simulink model "Environment"  (R2014b)
settings: Solver=ode45  StartTime=0.0  StopTime=10.0  RelTol=1e-3
model workspace (MATLAB code in the model file):
  | switch(Env)
  |    case 'Pikes Peak'
  |       load Evn_Pikes_Peak;
  |    case 'IOM'
  |       load Evn_IOM;
  |    otherwise
  |       load Environment
  | end
undefined symbols (not defined in the file): altx, alty, g, L, M, P0, R, Rcx, Rcy, T0
settings Model: Creator=Nathan  LastModifiedBy=Nathan
settings DebuggingCC: UnderspecifiedInitializationDetection=Classic  MergeDetectMultiDrivingBlocksExec=none  StateNameClashWarn=warning

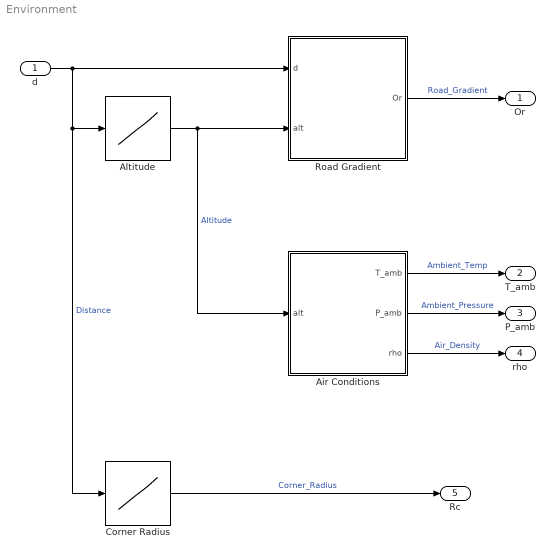
== system Environment ==
  d : Inport
  Air Conditions : Subsystem
  Altitude : Lookup_n-D  NumberOfTableDimensions=1  BreakpointsForDimension1=altx  Table=alty  ExtrapMethod=Clip  DiagnosticForOutOfRangeInput=Warning  UseLastTableValue=on  RndMeth=Simplest  InputSameDT=on
  Corner Radius : Lookup_n-D  NumberOfTableDimensions=1  BreakpointsForDimension1=Rcx  Table=Rcy  ExtrapMethod=Clip  DiagnosticForOutOfRangeInput=Warning  UseLastTableValue=on  RndMeth=Simplest  InputSameDT=on
  Road Gradient : Subsystem
  Or : Outport
  T_amb : Outport  Port=2
  P_amb : Outport  Port=3
  rho : Outport  Port=4
  Rc : Outport  Port=5
  wires:
  d/1 -> Road Gradient/1(d), Corner Radius/1, Altitude/1  "Distance"
  Road Gradient/1(Or) -> Or/1  "Road_Gradient"
  Altitude/1 -> Air Conditions/1(alt), Road Gradient/2(alt)  "Altitude"
  Air Conditions/1("T_amb ") -> T_amb/1  "Ambient_Temp"
  Air Conditions/2(P_amb) -> P_amb/1  "Ambient_Pressure"
  Air Conditions/3(rho) -> rho/1  "Air_Density"
  Corner Radius/1 -> Rc/1  "Corner_Radius"

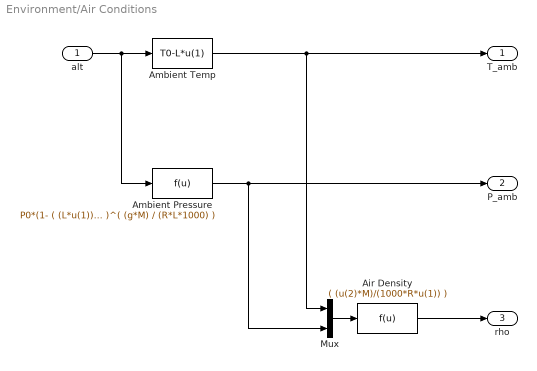
== system Environment/Air Conditions ==
  alt : Inport
  Air Density : Fcn  Expr=( (u(2)*M)/(1000*R*u(1)) )
  Ambient Pressure : Fcn  Expr=P0*(1- ( (L*u(1))/(T0) ) )^( (g*M) / (R*L*1000) )
  Ambient Temp : Fcn  Expr=T0-L*u(1)
  Mux : Mux  Inputs=2
  "T_amb " : Outport
  P_amb : Outport  Port=2
  rho : Outport  Port=3
  wires:
  alt/1 -> Ambient Pressure/1, Ambient Temp/1
  Ambient Temp/1 -> Mux/1, "T_amb "/1
  Ambient Pressure/1 -> Mux/2, P_amb/1
  Mux/1 -> Air Density/1
  Air Density/1 -> rho/1

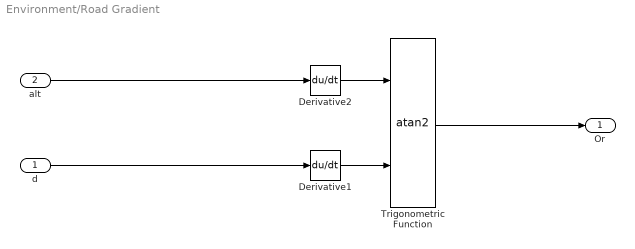
== system Environment/Road Gradient ==
  d : Inport
  alt : Inport  Port=2
  Derivative1 : Derivative
  Derivative2 : Derivative
  Trigonometric Function : Trigonometry  Operator=atan2
  Or : Outport
  wires:
  alt/1 -> Derivative2/1
  Trigonometric Function/1 -> Or/1
  Derivative1/1 -> Trigonometric Function/2
  d/1 -> Derivative1/1
  Derivative2/1 -> Trigonometric Function/1
